simulink model "tremore"  (R2020a)
settings: Solver=VariableStepAuto  StartTime=0.0  StopTime=10  MaxStep=1e-3  RelTol=1e-3
values from neighbouring files (symbols this model uses):
  g = 9.81    [dati_tesi_modellosimulink.m]
  L = 0.3    [dati_tesi_modellosimulink.m]
  Lc = L/2    (= 0.15)    [dati_tesi_modellosimulink.m]
  M = 4    [dati_tesi_modellosimulink.m]
  wc = 10*2*pi    (= 62.8318530718)    [dati_tesi_modellosimulink.m]
libraries: fuzblock x6, simulink x5, simulink_extras x1
settings Model: Creator=laura  LastModifiedBy=laura

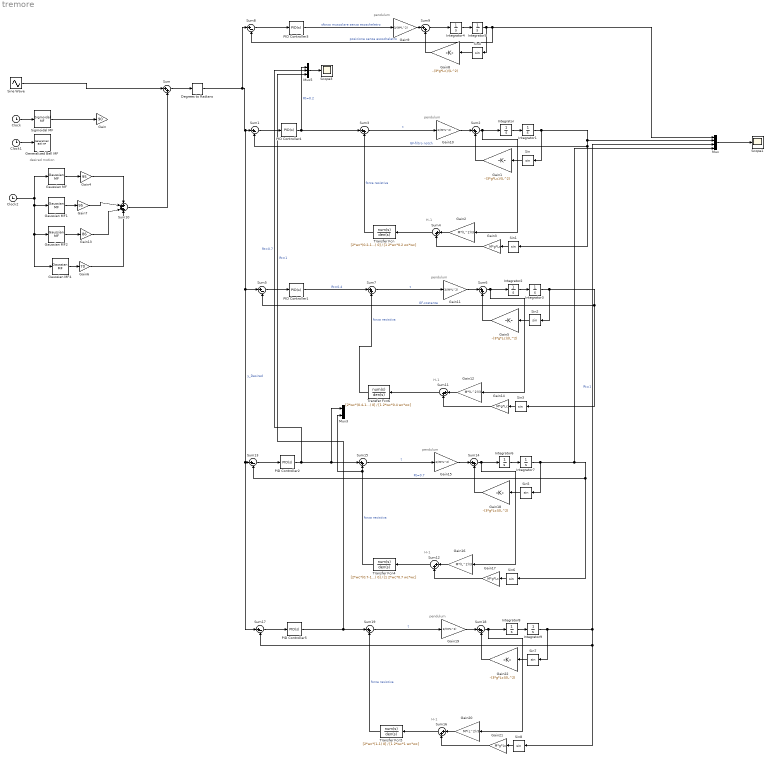
== system tremore ==
  note: pendulum
  note: H-1
  note: pendulum
  note: desired motion
  note: H-1
  note: pendulum
  note: pendulum
  note: H-1
  note: pendulum
  note: H-1
  Clock : Clock
  Clock1 : Clock
  Clock2 : Clock
  Degrees to Radians : simulink_extras/Transformations/Degrees to Radians
  Gain : Gain  Gain=90
  Gain{1,5,8,18,22} (5 alike) : Gain  Gain=-(3*g*Lc)/(L^2)
  Gain{9..11,15,19} (5 alike) : Gain  Gain=3/(M*L^2)
  Gain{2,12,16,20} (4 alike) : Gain  Gain=M*(L^2)/3
  Gain13 : Gain  Gain=86
  Gain{3,14,17,21} (4 alike) : Gain  Gain=M*g*Lc
  Gain4 : Gain  Gain=95
  Gain6 : Gain  Gain=70
  Gain7 : Gain  Gain=95
  Gaussian MF : fuzblock/Membership  Functions/Gaussian MF  sigma=0.4  mu=1.78
      settings: SourceProductBaseCode=FL
  Gaussian MF1 : fuzblock/Membership  Functions/Gaussian MF  sigma=0.4  mu=7
      settings: SourceProductBaseCode=FL
  Gaussian MF2 : fuzblock/Membership  Functions/Gaussian MF  sigma=0.38  mu=3.42
      settings: SourceProductBaseCode=FL
  Gaussian MF4 : fuzblock/Membership  Functions/Gaussian MF  sigma=0.32  mu=2.63
      settings: SourceProductBaseCode=FL
  Generalized Bell MF : fuzblock/Membership  Functions/Generalized Bell MF  a=1.5  b=4  c=6
      settings: SourceProductBaseCode=FL
  Integrator{,1..9} (10 alike) : Integrator
  Mux : Mux
  Mux3 : Mux  Inputs=2
  Mux5 : Mux  Inputs=3
  PID Controller{1..5} (5 alike) : simulink/Continuous/PID Controller  Controller=PID  Form=Parallel  TimeDomain=Continuous-time  UseExternalTs=off  SampleTime=-1  IntegratorMethod=Forward Euler  FilterMethod=Forward Euler  ControllerParametersSource=internal  P=20.396  I=105.7651  D=6.3413  UseFilter=on  N=150.7964  TunerSelectOption=Transfer Function Based (PID Tuner App)  InitialConditionSource=internal  InitialConditionForIntegrator=0  InitialConditionForFilter=0  DifferentiatorICPrevScaledInput=0  ExternalReset=none  TrackingMode=off  Kt=1  LimitOutput=off  UpperSaturationLimit=inf  LowerSaturationLimit=-inf  LinearizeAsGain=on  AntiWindupMode=none  Kb=1  POutMin=[]  POutMax=[]  IOutMin=[]  IOutMax=[]  DOutMin=[]  DOutMax=[]  NOutMin=[]  NOutMax=[]  SumOutMin=[]  SumOutMax=[]  SaturationOutMin=[]  SaturationOutMax=[]  PParamMin=[]  PParamMax=[]  IParamMin=[]  IParamMax=[]  DParamMin=[]  DParamMax=[]  NParamMin=[]  NParamMax=[]  KbParamMin=[]  KbParamMax=[]  KtParamMin=[]  KtParamMax=[]  KbOutMin=[]  KbOutMax=[]  KtOutMin=[]  KtOutMax=[]  IntegratorOutMin=[]  IntegratorOutMax=[]  FilterOutMin=[]  FilterOutMax=[]  SumI1OutMin=[]  SumI1OutMax=[]  SumI2OutMin=[]  SumI2OutMax=[]  SumI3OutMin=[]  SumI3OutMax=[]  SumI4OutMin=[]  SumI4OutMax=[]  SumDOutMin=[]  SumDOutMax=[]  DifferentiatorOutMin=[]  DifferentiatorOutMax=[]  FilterDiffOutCoefMin=[]  FilterDiffOutCoefMax=[]  ReciprocalOutMin=[]  ReciprocalOutMax=[]  SumDenOutMin=[]  SumDenOutMax=[]  SumNumOutMin=[]  SumNumOutMax=[]  DivideOutMin=[]  DivideOutMax=[]  UdiffTsProdOutMin=[]  UdiffTsProdOutMax=[]  NTsProdOutMin=[]  NTsProdOutMax=[]  UintegralTsProdOutMin=[]  UintegralTsProdOutMax=[]  UngainTsProdOutMin=[]  UngainTsProdOutMax=[]  IntegratorContinuousStateAttributes=''  IntegratorStateMustResolveToSignalObject=off  IntegratorRTWStateStorageClass=Auto  FilterContinuousStateAttributes=''  FilterStateMustResolveToSignalObject=off  FilterRTWStateStorageClass=Auto  ParallelPVariant=InternalParameters  IdealPVariant=Disabled  IVariant=InternalParameters  DVariant=InternalParameters  IntegratorVariant=Continuous  SatVariant=Disabled  AWVariant=Passthrough  PCopyVariant=Disabled  TRVariant=Disabled  FdbkBlocksVariant=Forward  IdealPFdbkVariant=Disabled  SatFdbkVariant=Disabled  DerivativeFilterVariant=ContFilter  NVariant=InternalParameters  NCopyVariant=Disabled  FilterICVariant=InternalICsFilter  IntegratorICVariant=InternalICs  ExternalResetVariant=Disabled  TRSumVariant=Passthrough  SumFdbkVariant=Disabled  SumVariant=Sum_PID  TsampFilterVariant=InternalTs  TsampNgainVariant=Passthrough  TsampIntegralVariant=Passthrough
  Scope1 : Scope
  Scope3 : Scope
  Sigmoidal MF : fuzblock/Membership  Functions/Sigmoidal MF  a=2  c=5
      settings: SourceProductBaseCode=FL
  Sin{,1..8} (9 alike) : Trigonometry
  Sine Wave : Sin  Amplitude=2.5  Frequency=10*2*pi  SampleTime=0
  Sum{,2..4,6..7,9,11..12,14..16,18..19} (14 alike) : Sum  Inputs=|++
  Sum{1,5,8,13,17} (5 alike) : Sum  Inputs=|+-
  Sum10 : Sum  Inputs=++++
  Transfer Fcn : TransferFcn  Numerator=[2*wc*(0.2-1) 0]  Denominator=[1 2*wc*0.2 wc*wc]
  Transfer Fcn4 : TransferFcn  Numerator=[2*wc*(0.7-1) 0]  Denominator=[1 2*wc*0.7 wc*wc]
  Transfer Fcn5 : TransferFcn  Numerator=[2*wc*(1-1) 0]  Denominator=[1 2*wc*1 wc*wc]
  Transfer Fcn6 : TransferFcn  Numerator=[2*wc*(0.4-1) 0]  Denominator=[1 2*wc*0.4 wc*wc]
  wires:
  Clock/1 -> Sigmoidal MF/1
  Sine Wave/1 -> Sum/1
  Sum/1 -> Degrees to Radians/1
  PID Controller3/1 -> Gain9/1  "sforzo muscolare senza esoscheletro"
  Integrator5/1 -> Mux/1, Sum8/2, Sin4/1  "posizione senza esoscheletro"
  Sum3/1 -> Gain10/1  "t"
  PID Controller4/1 -> Mux5/1, Sum3/1  "Rt=0.2"
  Sum8/1 -> PID Controller3/1
  Sum9/1 -> Integrator4/1
  Gain9/1 -> Sum9/1
  Integrator1/1 -> Sin/1, Sin1/1, Sum1/2, Mux/2  "GF-filtro notch"
  Gain1/1 -> Sum2/2
  Sum1/1 -> PID Controller4/1
  Sin/1 -> Gain1/1
  Sin1/1 -> Gain3/1
  Sin4/1 -> Gain8/1
  Mux/1 -> Scope1/1
  Gain3/1 -> Sum4/2
  Gain10/1 -> Sum2/1
  Integrator/1 -> Integrator1/1
  Gain8/1 -> Sum9/2
  Integrator4/1 -> Integrator5/1
  Sum2/1 -> Integrator/1, Gain2/1
  Gain2/1 -> Sum4/1
  Sum4/1 -> Transfer Fcn/1
  Transfer Fcn/1 -> Sum3/2  "forza resistiva"
  Clock1/1 -> Generalized Bell MF/1
  Gain4/1 -> Sum10/1
  Gaussian MF4/1 -> Gain6/1
  Clock2/1 -> Gaussian MF/1, Gaussian MF4/1, Gaussian MF2/1, Gaussian MF1/1
  Gaussian MF2/1 -> Gain13/1
  Gain13/1 -> Sum10/3
  Gain6/1 -> Sum10/4
  Gaussian MF/1 -> Gain4/1
  Gaussian MF1/1 -> Gain7/1
  Gain7/1 -> Sum10/2
  Transfer Fcn6/1 -> Sum7/2  "forza resistiva"
  Sum11/1 -> Transfer Fcn6/1
  Gain5/1 -> Sum6/2
  Sum5/1 -> PID Controller1/1
  Integrator2/1 -> Integrator3/1
  Gain12/1 -> Sum11/1
  Sin2/1 -> Gain5/1
  Gain14/1 -> Sum11/2
  Integrator3/1 -> Sin2/1, Sum5/2, Sin3/1  "GF-costante"
  Sin3/1 -> Gain14/1
  Gain11/1 -> Sum6/1
  PID Controller1/1 -> Sum7/1  "Rt=0.4"
  Sum6/1 -> Integrator2/1, Gain12/1
  Sum7/1 -> Gain11/1  "t"
  Degrees to Radians/1 -> Sum8/1, Sum17/1, Sum13/1, Sum5/1, Sum1/1  "y_Desired"
  Sum14/1 -> Integrator6/1, Gain16/1
  Sum15/1 -> Gain15/1  "t"
  Integrator7/1 -> Sin5/1, Mux/4, Sum13/2, Sin6/1  "Rt=0.7"
  Sin6/1 -> Gain17/1
  Gain15/1 -> Sum14/1
  Sin5/1 -> Gain18/1
  Gain16/1 -> Sum12/1
  Gain17/1 -> Sum12/2
  Integrator6/1 -> Integrator7/1
  Transfer Fcn4/1 -> Mux3/2, Sum15/2  "forza resistiva"
  Sum12/1 -> Transfer Fcn4/1
  PID Controller2/1 -> Mux5/2, Mux3/1, Sum15/1  "Rt=0.7"
  Gain18/1 -> Sum14/2
  Sum13/1 -> PID Controller2/1
  Sigmoidal MF/1 -> Gain/1
  Mux5/1 -> Scope3/1
  Sum19/1 -> Gain19/1  "t"
  Gain21/1 -> Sum16/2
  Gain20/1 -> Sum16/1
  Sin7/1 -> Gain22/1
  Gain19/1 -> Sum18/1
  Sum18/1 -> Integrator8/1, Gain20/1
  Sin8/1 -> Gain21/1
  Integrator8/1 -> Integrator9/1
  Sum16/1 -> Transfer Fcn5/1
  Integrator9/1 -> Sin7/1, Sin8/1, Sum17/2, Mux/3  "Rt=1"
  Transfer Fcn5/1 -> Sum19/2  "forza resistiva"
  Gain22/1 -> Sum18/2
  PID Controller5/1 -> Mux5/3, Sum19/1  "Rt=1"
  Sum17/1 -> PID Controller5/1
  Sum10/1 -> Sum/2
